simulink model "TEST_Wind"  (R2019b)
settings: Solver=ode1  StartTime=0.0  StopTime=15  FixedStep=1/250  RelTol=1e-3
undefined symbols (not defined in the file or in its folder): F, Light, MIL
libraries: aerolibwind2 x2
settings Model: Creator=sl  LastModifiedBy=sl

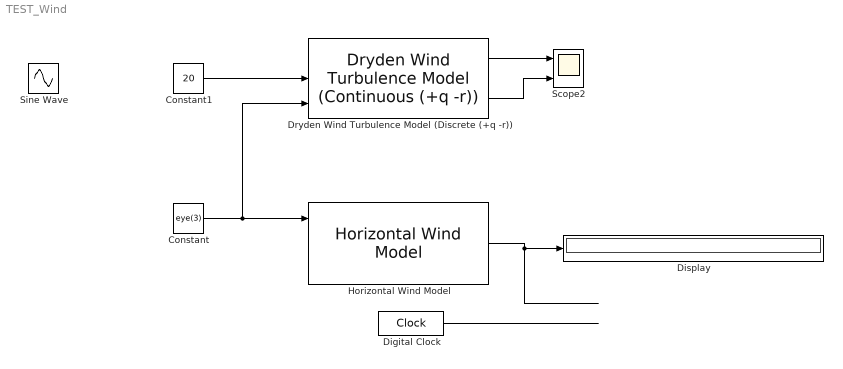
== system TEST_Wind ==
  Constant : Constant  Value=eye(3)
  Constant1 : Constant  Value=20
  Digital Clock : DigitalClock
  Display : Display
  Dryden Wind Turbulence Model (Discrete (+q -r)) : aerolibwind2/Dryden Wind Turbulence Model  (Continuous (+q -r))  units=Metric (MKS)  spec=MIL-F-8785C  model=Discrete Dryden (+q -r)  W20=10  Wdeg=0  TurbProb=10^-2 - Light  L_high=533.4  Wingspan=100  ts=1/250  Seed=[23341 23342 23343 23344]  T_on=on
      settings: SourceProductName=Aerospace Blockset
  Horizontal Wind Model : aerolibwind2/Horizontal Wind Model  units=Metric (MKS)  Vw_source=External  Vwind=5  W_source=External  Wdeg=0
      settings: SourceProductName=Aerospace Blockset  SourceProductBaseCode=AE
  Scope2 : Scope  NumInputPorts=2
  Sine Wave : Sin  SampleTime=0
  wires:
  Horizontal Wind Model/1 -> Display/1
  Constant/1 -> Horizontal Wind Model/1, Dryden Wind Turbulence Model (Discrete (+q -r))/3
  Digital Clock/1 -> ?
  Constant1/1 -> Dryden Wind Turbulence Model (Discrete (+q -r))/2
  Dryden Wind Turbulence Model (Discrete (+q -r))/1 -> Scope2/1
  Dryden Wind Turbulence Model (Discrete (+q -r))/2 -> Scope2/2
